simulink model "thingspeak_task"  (Simulink 3.00)
undefined symbols (not defined in the file): application, json
libraries: stringlib x4, mathlib x3, speclib x1

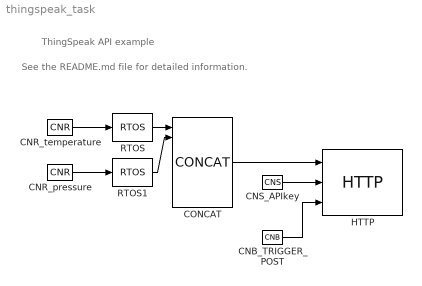
== system thingspeak_task ==
  note: See the README.md file for detailed information.
  note: ThingSpeak API example
  CNB_TRIGGER_POST : mathlib/CNB  YCN=off
  CNR_pressure : mathlib/CNR  ycn=105
  CNR_temperature : mathlib/CNR  ycn=9.81
  CNS_APIkey : stringlib/CNS  scv=YourThingspeakAPIkey  nmax=0
  CONCAT : stringlib/CONCAT  ptrn="{ \"field1\": %1, \"field2\": %2 }"  nmax=0
  HTTP : speclib/HTTP  url=https://api.thingspeak.com/update.json?api_key=  method=2  VERIFY=off  postmime=application/json  acceptmime=application/json  timeout=5  BLOCKING=off  nmax=0  postmax=256  datamax=1024
  RTOS : stringlib/RTOS  prec=3  mode=2
  RTOS1 : stringlib/RTOS  prec=0  mode=2
  wires:
  CNB_TRIGGER_POST/1 -> HTTP/3
  CNR_pressure/1 -> RTOS1/1
  CNR_temperature/1 -> RTOS/1
  CNS_APIkey/1 -> HTTP/2
  CONCAT/1 -> HTTP/1
  RTOS/1 -> CONCAT/1
  RTOS1/1 -> CONCAT/2
